simulink model "total_sem subsystem"  (R2020a)
settings: Solver=VariableStepAuto  StartTime=0.0  StopTime=10.0  RelTol=1e-3
values from neighbouring files (symbols this model uses):
  G = 9.8    [main_ficheiros separados.m]    (also in main_graficos_juntos_3a3.m)
  Kt = 3.575e-5    (= 3.575e-05)    [main_ficheiros separados.m]    (also in main_graficos_juntos_3a3.m)
  M = 1    [main_ficheiros separados.m]    (also in main_graficos_juntos_3a3.m)
  omega_0 = sqrt(G*M/Kt)    [main_ficheiros separados.m]    (also in main_graficos_juntos_3a3.m)
  u_0 = omega_0    [main_ficheiros separados.m]    (also in main_graficos_juntos_3a3.m)
  Z0 = 2    [main_ficheiros separados.m]    (also in main_graficos_juntos_3a3.m)
undefined symbols (not defined in the file or in its folder): i
settings Model: Creator=josem  LastModifiedBy=josem

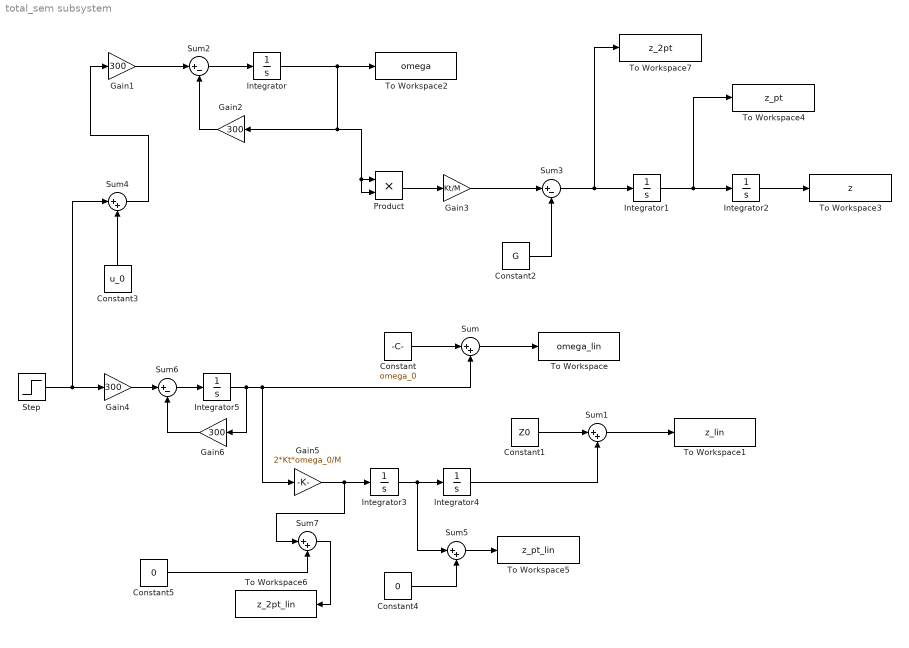
== system total_sem subsystem ==
  Constant : Constant  Value=omega_0
  Constant1 : Constant  Value=Z0
  Constant2 : Constant  Value=G
  Constant3 : Constant  Value=u_0
  Constant4 : Constant  Value=0
  Constant5 : Constant  Value=0
  Gain{1..2,4,6} (4 alike) : Gain  Gain=300
  Gain3 : Gain  Gain=Kt/M
  Gain5 : Gain  Gain=2*Kt*omega_0/M
  Integrator : Integrator  InitialCondition=omega_0  LimitOutput=on  UpperSaturationLimit=3*omega_0  LowerSaturationLimit=0
  Integrator{1,3..5} (4 alike) : Integrator
  Integrator2 : Integrator  InitialCondition=Z0
  Product : Product
  Step : Step  After=u(i)-u_0  SampleTime=0
  Sum{,1,4..5,7} (5 alike) : Sum  Inputs=|++
  Sum2 : Sum  Inputs=|+-
  Sum3 : Sum  Inputs=|+-
  Sum6 : Sum  Inputs=|+-
  To Workspace : ToWorkspace  VariableName=omega_lin  SaveFormat=Structure With Time  SampleTime=-1
  To Workspace1 : ToWorkspace  VariableName=z_lin  SaveFormat=Structure With Time  SampleTime=-1
  To Workspace2 : ToWorkspace  VariableName=omega  SaveFormat=Structure With Time  SampleTime=-1
  To Workspace3 : ToWorkspace  VariableName=z  SaveFormat=Structure With Time  SampleTime=-1
  To Workspace4 : ToWorkspace  VariableName=z_pt  SaveFormat=Structure With Time  SampleTime=-1
  To Workspace5 : ToWorkspace  VariableName=z_pt_lin  SaveFormat=Structure With Time  SampleTime=-1
  To Workspace6 : ToWorkspace  VariableName=z_2pt_lin  SaveFormat=Structure With Time  SampleTime=-1
  To Workspace7 : ToWorkspace  VariableName=z_2pt  SaveFormat=Structure With Time  SampleTime=-1
  wires:
  Constant/1 -> Sum/1
  Sum1/1 -> To Workspace1/1
  Constant1/1 -> Sum1/1
  Sum/1 -> To Workspace/1
  Integrator5/1 -> Gain6/1, Sum/2, Gain5/1
  Integrator/1 -> Product/2, Product/1, Gain2/1, To Workspace2/1
  Gain3/1 -> Sum3/1
  Integrator2/1 -> To Workspace3/1
  Gain2/1 -> Sum2/2
  Integrator1/1 -> To Workspace4/1, Integrator2/1
  Sum3/1 -> To Workspace7/1, Integrator1/1
  Product/1 -> Gain3/1
  Constant2/1 -> Sum3/2
  Sum2/1 -> Integrator/1
  Gain1/1 -> Sum2/1
  Constant3/1 -> Sum4/2
  Sum4/1 -> Gain1/1
  Step/1 -> Gain4/1, Sum4/1
  Gain5/1 -> Sum7/1, Integrator3/1
  Integrator4/1 -> Sum1/2
  Integrator3/1 -> Sum5/1, Integrator4/1
  Constant4/1 -> Sum5/2
  Sum5/1 -> To Workspace5/1
  Gain4/1 -> Sum6/1
  Sum6/1 -> Integrator5/1
  Gain6/1 -> Sum6/2
  Constant5/1 -> Sum7/2
  Sum7/1 -> To Workspace6/1
